simulink model "SPMSM_back_EMF_Observer_SMO_Trigger"  (R2022b)
settings: Solver=VariableStepAuto  StartTime=0.0  StopTime=4  FixedStep=1e-7  MaxStep=1e-7  RelTol=1e-6
undefined symbols (not defined in the file): DiscIntNeverNeededParam
libraries: slpidlib x4, dspsigops x4, dsparch4 x3, simulink x2, spsDCVoltageSourceLib x1, spsPermanentMagnetSynchronousMachineLib x1, dspstat3 x1, spsUniversalBridgeLib x1, spspowerguiLib x1
settings Model: Creator=SSC  LastModifiedBy=SSC

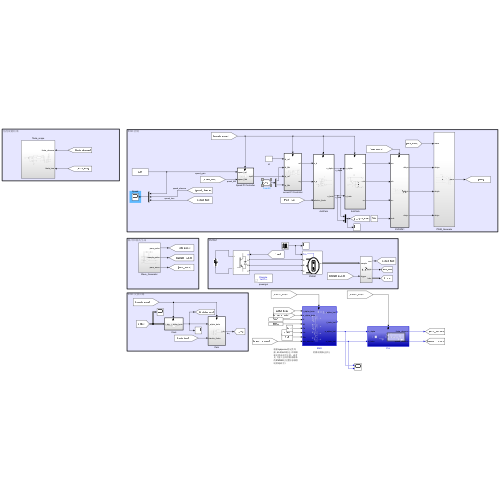
[thumbnail: Simulink's stored preview of the top-level diagram]
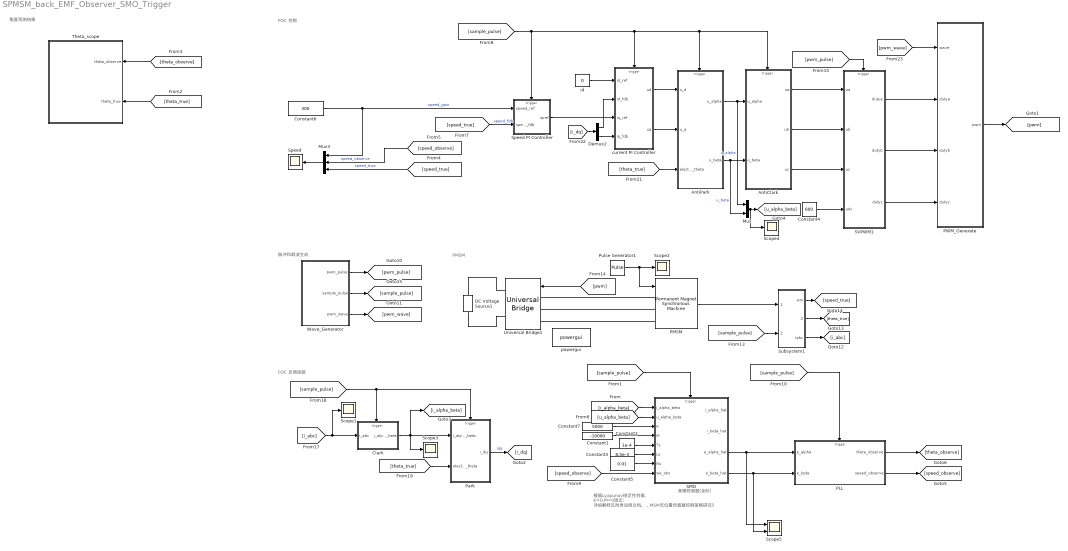
== system SPMSM_back_EMF_Observer_SMO_Trigger ==
  note: 根据Lyapunov稳定性判据, K>0,M<0稳定; 详细解释见附录说明文档。或者见《基于全阶滑模观测器的IPMSM无位置传感器控制策略研究》
  note: 滑模观测器(全阶)
  note: 角度观测结果
  note: FOC 控制
  note: FOC 反馈回路
  note: 脉冲和载波生成
  note: PMSM
  AntiClark : Subsystem
  AntiPark : Subsystem
  Clark : Subsystem
  Constant1 : Constant  Value=-10000
  Constant2 : Constant  Value=1e-4
  Constant3 : Constant  Value=8.5e-3
  Constant4 : Constant  Value=600
  Constant5 : Constant  Value=0.91
  Constant6 : Constant  Value=300
  Constant7 : Constant  Value=5000
  DC Voltage Source1 : spsDCVoltageSourceLib/DC Voltage Source  Amplitude=600  Measurements=None
  Demux2 : Demux  Outputs=2
  Mux : Mux  Inputs=2
  Mux3 : Mux  Inputs=3
  PLL : Subsystem  TreatAsAtomicUnit=on
  PMSM : spsPermanentMagnetSynchronousMachineLib/Permanent Magnet Synchronous Machine  NbPhases=3  FluxDistribution=Sinusoidal  RotorType=Round  MechanicalLoad=Torque Tm  PresetModel=No  ShowDetailedParameters=on  MeasurementBus=off  Resistance=0.91  Inductance=8.5e-3  dqInductances=[0.00396,0.00396]  La=8.5e-3  MachineConstant=Flux linkage established by magnets (V.s)  Flux=0.446  VoltageCst=161.7909  TorqueCst=1.338  Flat=120  Mechanical=[0.074 0.008 2 0]  PolePairs=4  InitialConditions=[300*2*pi/60,0,0,0]  InitialConditions5ph=[0 0 0 0 0 0]  RefAngle=Aligned with phase A axis (original Park)  IterativeDiscreteModel=Trapezoidal non iterative  TsBlock=-1  TsPowergui=0
  PWM_Generate : Subsystem
  Park : Subsystem
  Pulse Generator1 : DiscretePulseGenerator  PulseType=Time based  Period=3  PulseWidth=33.3  PhaseDelay=2.5
  SMO : Subsystem  TreatAsAtomicUnit=on
  SVPWM1 : Subsystem
  Scope{1..4} (4 alike) : Scope
  Scope5 : Scope  NumInputPorts=2
  Speed : Scope
  Speed PI Controller : Subsystem  TreatAsAtomicUnit=on
  Subsystem1 : Subsystem
  Theta_scope : Subsystem
  Universal Bridge1 : spsUniversalBridgeLib/Universal Bridge  Arms=3  SnubberResistance=1e5  SnubberCapacitance=inf  Device=IGBT / Diodes  Ron=1e-3  Lon=0  ForwardVoltages="[  0  0  ]"  ForwardVoltage=0  GTOparameters=[ 10e-6 , 20e-6 ]  IGBTparameters=[ 1e-6 , 2e-6 ]  Measurements=None  Measurements_2=None  converterType=Rectifier
  Wave_Generator : Subsystem
  current PI Controller : Subsystem
  id : Constant  Value=0
  powergui : spspowerguiLib/powergui  Priority=1  SimulationMode=Discrete  SampleTime=1e-7  frequency=60  Iterations=50  frequencyindice=0  Pbase=100e6  ErrMax=1e-4  UnitsV=kV  UnitsW=MW  buscounter=0  FunctionMessages=off  echomessages=off  EnableUseOfTLC=off  CurrentSourceSwitches=off  DisableSnubberDevices=off  DisableRonSwitches=off  DisableVfSwitches=off  DisplayEquations=off  AutomaticDiscreteSolvers=off  SolverType=Tustin/Backward Euler (TBE)  Interpol=off  ExternalGateDelay=off  methode=off  Ts=100  x0status=blocks  SPID=on  SwTol=0  HookPort=off  NonlinearTolerance=1e-4  nMaxIteration=100  ContinueOnMaxIteration=off  RestoreLinks=warning  ResistiveCurrentMeasurement=off  Frange=[0:2:500]  Ylog=off  Xlog=on  ShowGrid=off  save=off  variable=ZData  structure=0  ZoomFFT=off  StartTime=0.0  cycles=1  DisplayStyle=1  fundamental=60  FreqAxis=off  MaxFrequency=1000  frequencyindicesteady=1  RmsSteady=1  display=off
  wires:
  PMSM/1 -> Subsystem1/1(sample)
  [pwm] -> Universal Bridge1/1
  Subsystem1/2(theta) -> [theta_true]
  Subsystem1/3(Iabc) -> [i_abc]
  Pulse Generator1/1 -> PMSM/1, Scope2/1
  Wave_Generator/1(pwm_pulse) -> [pwm_pulse]
  Wave_Generator/2(sample_pulse) -> [sample_pulse]
  Wave_Generator/3(pwm_wave) -> [pwm_wave]
  Subsystem1/1(wm) -> [speed_true]
  [sample_pulse] -> Subsystem1/2(trigger)
  [sample_pulse] -> Park/Trigger, Clark/Trigger
  [theta_true] -> Park/2(electric_theta)
  Park/1(i_dq) -> [i_dq]  "idq"
  [i_abc] -> Scope1/1, Clark/1(i_abc)
  Clark/1(i_alpha_beta) -> [i_alpha_beta], Scope3/1, Park/1(i_alpha_beta)
  AntiClark/3(uc) -> SVPWM1/3(uc)
  [pwm_pulse] -> SVPWM1/Trigger
  AntiClark/1(ua) -> SVPWM1/1(ua)
  AntiClark/2(ub) -> SVPWM1/2(ub)
  SVPWM1/2(dutyb) -> PWM_Generate/3(dutyb)
  Constant4/1 -> SVPWM1/4(udc)
  SVPWM1/1(dutya) -> PWM_Generate/2(dutya)
  PWM_Generate/1(pwm) -> [pwm]
  SVPWM1/3(dutyc) -> PWM_Generate/4(dutyc)
  [pwm_wave] -> PWM_Generate/1(wave)
  [i_dq] -> Demux2/1
  id/1 -> current PI Controller/1(id_ref)
  Demux2/1 -> current PI Controller/2(id_fdb)
  Demux2/2 -> current PI Controller/4(iq_fdb)
  Speed PI Controller/1(iqref) -> current PI Controller/3(iq_ref)
  current PI Controller/1(ud) -> AntiPark/1(u_d)
  [theta_true] -> AntiPark/3(electric_theta)
  [speed_true] -> Speed PI Controller/2(speed_fdb)  "speed_fdb"
  current PI Controller/2(uq) -> AntiPark/2(u_q)
  AntiPark/1(u_alpha) -> Mux/1, AntiClark/1(u_alpha)  "u_alpha"
  AntiPark/2(u_beta) -> Mux/2, AntiClark/2(u_beta)  "u_beta"
  [theta_true] -> Theta_scope/2(theta_true)
  [theta_observe] -> Theta_scope/1(theta_observe)
  Constant6/1 -> Speed PI Controller/1(speed_ref), Mux3/1  "speed_gain"
  [speed_true] -> Mux3/3  "speed_true"
  [speed_observe] -> Mux3/2  "speed_observe"
  Mux3/1 -> Speed/1
  [sample_pulse] -> AntiClark/Trigger, AntiPark/Trigger, current PI Controller/Trigger, Speed PI Controller/Trigger
  Mux/1 -> Scope4/1, [u_alpha_beta]
  [i_alpha_beta] -> SMO/1(i_alpha_beta)
  [u_alpha_beta] -> SMO/2(u_alpha_beta)
  Constant7/1 -> SMO/3(K)
  Constant1/1 -> SMO/4(M)
  Constant2/1 -> SMO/5(Ts)
  Constant3/1 -> SMO/6(Ls)
  Constant5/1 -> SMO/7(Rs)
  [sample_pulse] -> SMO/Trigger
  SMO/3(e_alpha_hat) -> PLL/1(e_alpha), Scope5/1
  SMO/4(e_beta_hat) -> PLL/2(e_beta), Scope5/2
  [sample_pulse] -> PLL/Trigger
  PLL/2(speed_observe) -> [speed_observe]
  PLL/1(theta_observe) -> [theta_observe]
  [speed_observe] -> SMO/8(we_obs)
  connections:
  PMSM/LConn2 -- Universal Bridge1/LConn2
  PMSM/LConn1 -- Universal Bridge1/LConn1
  PMSM/LConn3 -- Universal Bridge1/LConn3
  Universal Bridge1/RConn1 -- DC Voltage Source1/RConn1
  DC Voltage Source1/LConn1 -- Universal Bridge1/RConn2

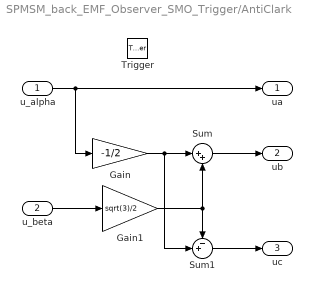
== system SPMSM_back_EMF_Observer_SMO_Trigger/AntiClark ==
  u_alpha : Inport
  u_beta : Inport  Port=2
  Trigger : TriggerPort  VariantControl=(inherit)
  Gain : Gain  Gain=-1/2
  Gain1 : Gain  Gain=sqrt(3)/2
  Sum : Sum  Inputs=|++
  Sum1 : Sum  Inputs=-+|
  ua : Outport
  ub : Outport  Port=2
  uc : Outport  Port=3
  wires:
  Sum1/1 -> uc/1
  Gain1/1 -> Sum1/1, Sum/2
  Sum/1 -> ub/1
  Gain/1 -> Sum/1, Sum1/2
  u_beta/1 -> Gain1/1
  u_alpha/1 -> ua/1, Gain/1

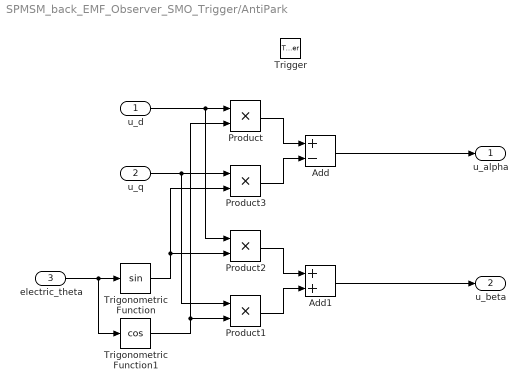
== system SPMSM_back_EMF_Observer_SMO_Trigger/AntiPark ==
  u_d : Inport
  u_q : Inport  Port=2
  electric_theta : Inport  Port=3
  Trigger : TriggerPort  VariantControl=(inherit)
  Add : Sum  Inputs=+-
  Add1 : Sum
  Product{,1..3} (4 alike) : Product
  Trigonometric Function : Trigonometry
  Trigonometric Function1 : Trigonometry  Operator=cos
  u_alpha : Outport
  u_beta : Outport  Port=2
  wires:
  electric_theta/1 -> Trigonometric Function1/1, Trigonometric Function/1
  u_d/1 -> Product2/1, Product/1
  Trigonometric Function1/1 -> Product/2, Product1/2
  u_q/1 -> Product1/1, Product3/1
  Trigonometric Function/1 -> Product2/2, Product3/2
  Product/1 -> Add/1
  Product3/1 -> Add/2
  Add/1 -> u_alpha/1
  Product2/1 -> Add1/1
  Product1/1 -> Add1/2
  Add1/1 -> u_beta/1

== system SPMSM_back_EMF_Observer_SMO_Trigger/Clark ==
  i_abc : Inport
  Trigger : TriggerPort  VariantControl=(inherit)
  Clark : Subsystem
  Demux : Demux  Outputs=3
  Mux6 : Mux  Inputs=2
  i_alpha_beta : Outport  VectorParamsAs1DForOutWhenUnconnected=off
  wires:
  Clark/2(I_beta) -> Mux6/2
  Mux6/1 -> i_alpha_beta/1
  Demux/3 -> Clark/3(I_c)
  Clark/1(I_alpha) -> Mux6/1
  i_abc/1 -> Demux/1
  Demux/2 -> Clark/2(I_b)
  Demux/1 -> Clark/1(I_a)

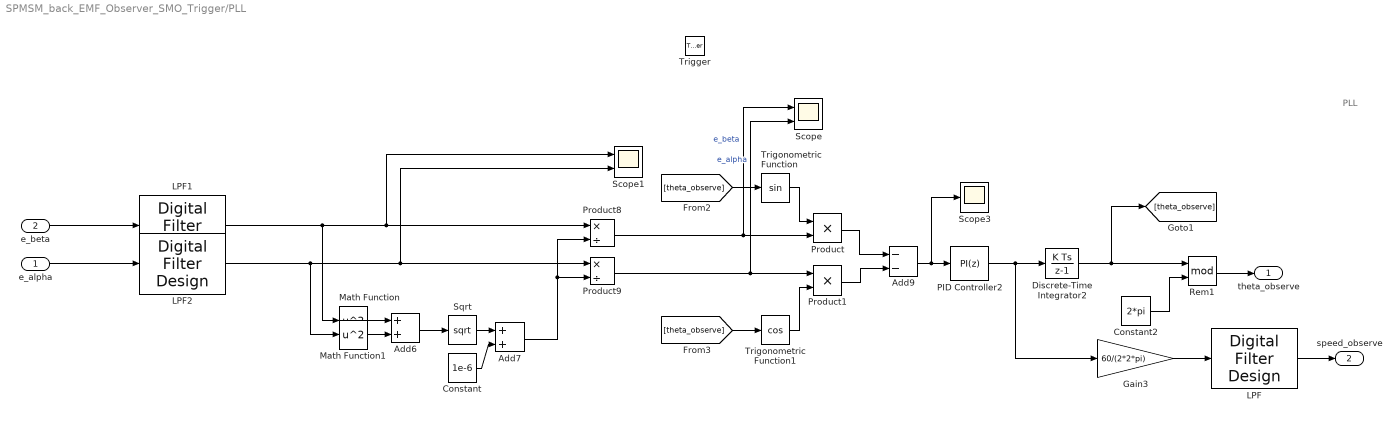
== system SPMSM_back_EMF_Observer_SMO_Trigger/PLL ==
  note: PLL
  e_alpha : Inport
  e_beta : Inport  Port=2
  Trigger : TriggerPort  VariantControl=(inherit)
  Add6 : Sum
  Add7 : Sum
  Add9 : Sum  Inputs=--
  Constant : Constant  Value=1e-6
  Constant2 : Constant  Value=2*pi
  Discrete-Time Integrator2 : DiscreteIntegrator  SampleTime=-1  ICPrevOutput=DiscIntNeverNeededParam  ICPrevScaledInput=DiscIntNeverNeededParam
  Gain3 : Gain  Gain=60/(2*2*pi)
  LPF : dsparch4/Digital Filter Design  mwdsp_browser_bugfix_var=off
  LPF1 : dsparch4/Digital Filter Design  mwdsp_browser_bugfix_var=off
  LPF2 : dsparch4/Digital Filter Design  mwdsp_browser_bugfix_var=off
  Math Function : Math  Operator=square
  Math Function1 : Math  Operator=square
  PID Controller2 : slpidlib/PID Controller  Controller=PI  Form=Parallel  TimeDomain=Discrete-time  UseExternalTs=off  SampleTime=-1  IntegratorMethod=Forward Euler  FilterMethod=Forward Euler  ControllerParametersSource=internal  P=10000  I=20000  UseKiTs=off  D=0  N=100  UseFilter=on  TunerSelectOption=Transfer Function Based (PID Tuner App)  InitialConditionSource=internal  InitialConditionForIntegrator=0  InitialConditionForFilter=0  DifferentiatorICPrevScaledInput=0  ExternalReset=none  TrackingMode=off  Kt=1  LimitOutput=off  SatLimitsSource=internal  UpperSaturationLimit=inf  LowerSaturationLimit=-inf  LinearizeAsGain=on  AntiWindupMode=none  Kb=1  LimitIntegrator=off  UpperIntegratorSaturationLimit=inf  LowerIntegratorSaturationLimit=-inf  POutMin=[]  POutMax=[]  IOutMin=[]  IOutMax=[]  DOutMin=[]  DOutMax=[]  NOutMin=[]  NOutMax=[]  SumOutMin=[]  SumOutMax=[]  SaturationOutMin=[]  SaturationOutMax=[]  PParamMin=[]  PParamMax=[]  IParamMin=[]  IParamMax=[]  DParamMin=[]  DParamMax=[]  NParamMin=[]  NParamMax=[]  KbParamMin=[]  KbParamMax=[]  KtParamMin=[]  KtParamMax=[]  KbOutMin=[]  KbOutMax=[]  KtOutMin=[]  KtOutMax=[]  IntegratorOutMin=[]  IntegratorOutMax=[]  FilterOutMin=[]  FilterOutMax=[]  SumI1OutMin=[]  SumI1OutMax=[]  SumI2OutMin=[]  SumI2OutMax=[]  SumI3OutMin=[]  SumI3OutMax=[]  SumI4OutMin=[]  SumI4OutMax=[]  SumDOutMin=[]  SumDOutMax=[]  DifferentiatorOutMin=[]  DifferentiatorOutMax=[]  FilterDiffOutCoefMin=[]  FilterDiffOutCoefMax=[]  ReciprocalOutMin=[]  ReciprocalOutMax=[]  SumDenOutMin=[]  SumDenOutMax=[]  SumNumOutMin=[]  SumNumOutMax=[]  DivideOutMin=[]  DivideOutMax=[]  UdiffTsProdOutMin=[]  UdiffTsProdOutMax=[]  NTsProdOutMin=[]  NTsProdOutMax=[]  UintegralTsProdOutMin=[]  UintegralTsProdOutMax=[]  UngainTsProdOutMin=[]  UngainTsProdOutMax=[]  ClampingZeroOutDataTypeStr=Inherit: Inherit via back propagation  ClampingZeroOutMin=[]  ClampingZeroOutMax=[]  FilterDenConstantOutDataTypeStr=Inherit: Inherit via back propagation  FilterDenConstantOutMin=[]  FilterDenConstantOutMax=[]  PCopyOutDataTypeStr=Inherit: Inherit via back propagation  PCopyOutMin=[]  PCopyOutMax=[]  NCopyOutDataTypeStr=Inherit: Inherit via back propagation  NCopyOutMin=[]  NCopyOutMax=[]  IntegratorContinuousStateAttributes=''  IntegratorStateMustResolveToSignalObject=off  IntegratorRTWStateStorageClass=Auto  FilterContinuousStateAttributes=''  FilterStateMustResolveToSignalObject=off  FilterRTWStateStorageClass=Auto  ParallelPVariant=InternalParameters  IdealPVariant=Disabled  IVariant=InternalParameters  DVariant=Disabled  IntegratorVariant=Discrete  SatVariant=Disabled  AWVariant=Passthrough  PCopyVariant=Disabled  TRVariant=Disabled  FdbkBlocksVariant=Forward  IdealPFdbkVariant=Disabled  SatFdbkVariant=Disabled  DerivativeFilterVariant=Disabled  NVariant=Disabled  NCopyVariant=Disabled_SignalSpec  FilterICVariant=Disabled  IntegratorICVariant=InternalICs  ExternalResetVariant=Disabled  TRSumVariant=Passthrough  SumFdbkVariant=Disabled  SumVariant=Sum_PI  TsampFilterVariant=InternalTs  TsampNgainVariant=Passthrough  TsampIntegralVariant=Passthrough  ExternalSaturationOutDataTypeStr=Inherit: Same as second input
  Product : Product
  Product1 : Product
  Product8 : Product  Inputs=*/
  Product9 : Product  Inputs=*/
  Rem1 : Math  Operator=mod
  Scope : Scope  NumInputPorts=2
  Scope1 : Scope  NumInputPorts=2
  Scope3 : Scope
  Sqrt : Sqrt
  Trigonometric Function : Trigonometry
  Trigonometric Function1 : Trigonometry  Operator=cos
  theta_observe : Outport
  speed_observe : Outport  Port=2  VectorParamsAs1DForOutWhenUnconnected=off
  wires:
  Trigonometric Function1/1 -> Product1/2
  [theta_observe] -> Trigonometric Function1/1
  Rem1/1 -> theta_observe/1
  Constant/1 -> Add7/2
  Product9/1 -> Scope/2, Product1/1  "e_alpha"
  Add7/1 -> Product8/2, Product9/2
  Sqrt/1 -> Add7/1
  Add6/1 -> Sqrt/1
  Math Function/1 -> Add6/1
  Math Function1/1 -> Add6/2
  LPF/1 -> speed_observe/1
  Gain3/1 -> LPF/1
  [theta_observe] -> Trigonometric Function/1
  Product1/1 -> Add9/2
  Discrete-Time Integrator2/1 -> Rem1/1, [theta_observe]
  Product8/1 -> Product/2, Scope/1  "e_beta"
  Constant2/1 -> Rem1/2
  Product/1 -> Add9/1
  Trigonometric Function/1 -> Product/1
  Add9/1 -> Scope3/1, PID Controller2/1
  PID Controller2/1 -> Gain3/1, Discrete-Time Integrator2/1
  e_beta/1 -> LPF1/1
  e_alpha/1 -> LPF2/1
  LPF1/1 -> Math Function/1, Product8/1, Scope1/1
  LPF2/1 -> Math Function1/1, Product9/1, Scope1/2

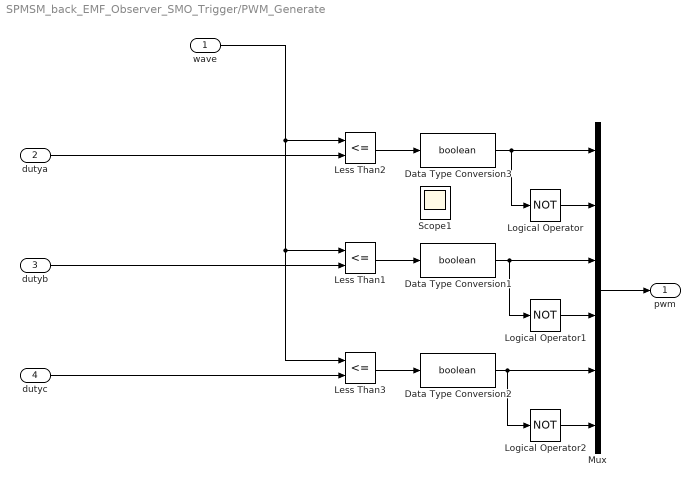
== system SPMSM_back_EMF_Observer_SMO_Trigger/PWM_Generate ==
  wave : Inport
  dutya : Inport  Port=2
  dutyb : Inport  Port=3
  dutyc : Inport  Port=4
  Data Type Conversion1 : DataTypeConversion  OutDataTypeStr=boolean  SaturateOnIntegerOverflow=off  RndMeth=Floor
  Data Type Conversion2 : DataTypeConversion  OutDataTypeStr=boolean  SaturateOnIntegerOverflow=off  RndMeth=Floor
  Data Type Conversion3 : DataTypeConversion  OutDataTypeStr=boolean  SaturateOnIntegerOverflow=off  RndMeth=Floor
  Less Than1 : RelationalOperator  Operator=<=  OutDataTypeStr=boolean  RndMeth=Simplest  InputSameDT=off
  Less Than2 : RelationalOperator  Operator=<=  OutDataTypeStr=boolean  RndMeth=Simplest  InputSameDT=off
  Less Than3 : RelationalOperator  Operator=<=  OutDataTypeStr=boolean  RndMeth=Simplest  InputSameDT=off
  Logical Operator : Logic  Operator=NOT  AllPortsSameDT=off  OutDataTypeStr=boolean
  Logical Operator1 : Logic  Operator=NOT  AllPortsSameDT=off  OutDataTypeStr=boolean
  Logical Operator2 : Logic  Operator=NOT  AllPortsSameDT=off  OutDataTypeStr=boolean
  Mux : Mux  Inputs=6
  Scope1 : Scope  NumInputPorts=2
  pwm : Outport
  wires:
  wave/1 -> Less Than3/1, Less Than1/1, Less Than2/1
  Less Than1/1 -> Data Type Conversion1/1
  Less Than2/1 -> Data Type Conversion3/1
  dutyb/1 -> Less Than1/2
  Less Than3/1 -> Data Type Conversion2/1
  dutya/1 -> Less Than2/2
  dutyc/1 -> Less Than3/2
  Data Type Conversion3/1 -> Logical Operator/1, Mux/1
  Logical Operator/1 -> Mux/2
  Data Type Conversion1/1 -> Logical Operator1/1, Mux/3
  Data Type Conversion2/1 -> Logical Operator2/1, Mux/5
  Logical Operator2/1 -> Mux/6
  Mux/1 -> pwm/1
  Logical Operator1/1 -> Mux/4

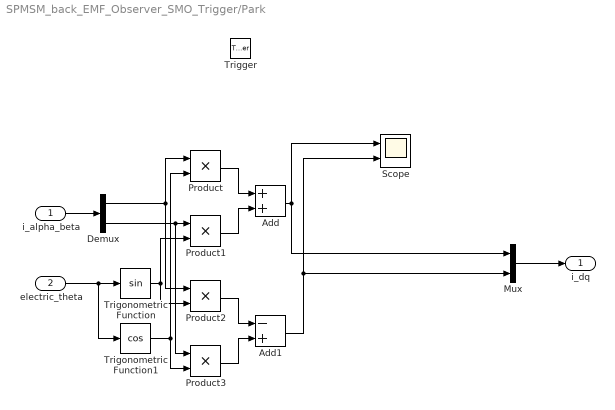
== system SPMSM_back_EMF_Observer_SMO_Trigger/Park ==
  i_alpha_beta : Inport
  electric_theta : Inport  Port=2
  Trigger : TriggerPort  VariantControl=(inherit)
  Add : Sum
  Add1 : Sum  Inputs=-+
  Demux : Demux  Outputs=2
  Mux : Mux  Inputs=2
  Product{,1..3} (4 alike) : Product
  Scope : Scope  NumInputPorts=2
  Trigonometric Function : Trigonometry
  Trigonometric Function1 : Trigonometry  Operator=cos
  i_dq : Outport
  wires:
  electric_theta/1 -> Trigonometric Function1/1, Trigonometric Function/1
  Trigonometric Function1/1 -> Product3/2, Product/2
  Demux/2 -> Product3/1, Product1/1
  Trigonometric Function/1 -> Product2/2, Product1/2
  Product/1 -> Add/1
  Product1/1 -> Add/2
  Product2/1 -> Add1/1
  Product3/1 -> Add1/2
  Demux/1 -> Product/1, Product2/1
  i_alpha_beta/1 -> Demux/1
  Mux/1 -> i_dq/1
  Add/1 -> Mux/1, Scope/1
  Add1/1 -> Mux/2, Scope/2

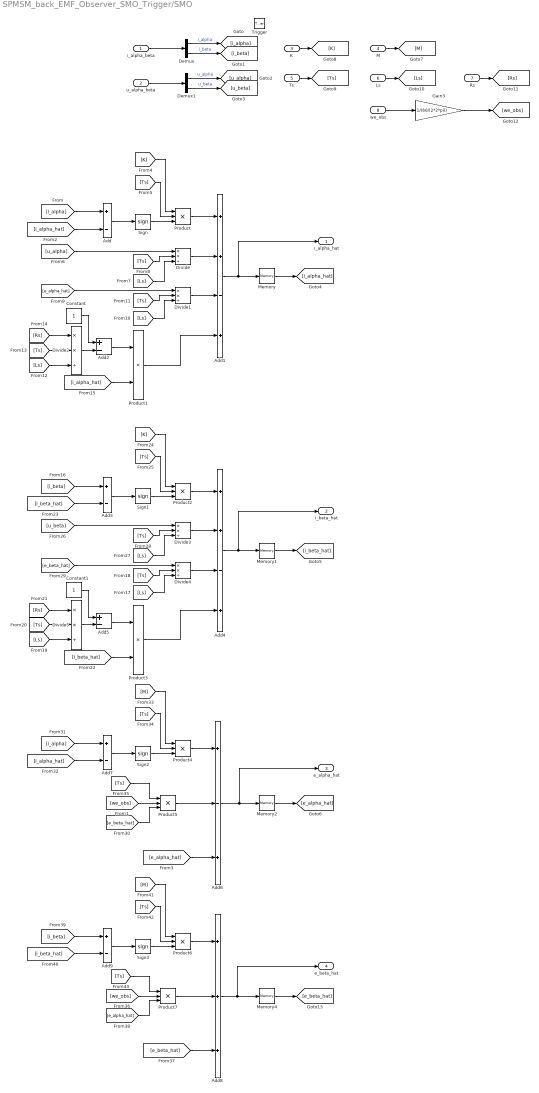
== system SPMSM_back_EMF_Observer_SMO_Trigger/SMO ==
  i_alpha_beta : Inport
  u_alpha_beta : Inport  Port=2
  K : Inport  Port=3
  M : Inport  Port=4
  Ts : Inport  Port=5
  Ls : Inport  Port=6
  Rs : Inport  Port=7
  we_obs : Inport  Port=8  LatchByDelayingOutsideSignal=on
  Trigger : TriggerPort  VariantControl=(inherit)
  Add{,2..3,5,7,9} (6 alike) : Sum  Inputs=+-
  Add1 : Sum  Inputs=++-+
  Add4 : Sum  Inputs=++-+
  Add6 : Sum  Inputs=+-+
  Add8 : Sum  Inputs=+++
  Constant : Constant
  Constant1 : Constant
  Demux : Demux  Outputs=2
  Demux1 : Demux  Outputs=2
  Divide{,1..5} (6 alike) : Product  Inputs=**/
  Gain3 : Gain  Gain=1/(60/(2*2*pi))
  Memory{,1..2,4} (4 alike) : Memory  InheritSampleTime=on
  Product{,2,4..7} (6 alike) : Product  Inputs=3
  Product1 : Product
  Product3 : Product
  Sign{,1..3} (4 alike) : Signum
  i_alpha_hat : Outport
  i_beta_hat : Outport  Port=2
  e_alpha_hat : Outport  Port=3
  e_beta_hat : Outport  Port=4
  wires:
  i_alpha_beta/1 -> Demux/1
  Demux/1 -> [i_alpha]  "i_alpha"
  Demux/2 -> [i_beta]  "i_beta"
  u_alpha_beta/1 -> Demux1/1
  Demux1/2 -> [u_beta]  "u_beta"
  Demux1/1 -> [u_alpha]  "u_alpha"
  [i_alpha] -> Add/1
  Memory/1 -> [i_alpha_hat]
  Memory1/1 -> [i_beta_hat]
  Memory2/1 -> [e_alpha_hat]
  [i_alpha_hat] -> Add/2
  Add/1 -> Sign/1
  Sign/1 -> Product/3
  K/1 -> [K]
  Ts/1 -> [Ts]
  [K] -> Product/1
  [Ts] -> Product/2
  Ls/1 -> [Ls]
  [Ls] -> Divide/3
  [u_alpha] -> Divide/1
  [Ts] -> Divide/2
  Product/1 -> Add1/1
  Divide/1 -> Add1/2
  [e_alpha_hat] -> Divide1/1
  [Ls] -> Divide1/3
  Divide1/1 -> Add1/3
  [Ts] -> Divide1/2
  Rs/1 -> [Rs]
  [Ls] -> Divide2/3
  [Ts] -> Divide2/2
  [Rs] -> Divide2/1
  Divide2/1 -> Add2/2
  Constant/1 -> Add2/1
  Add2/1 -> Product1/1
  [i_alpha_hat] -> Product1/2
  Product1/1 -> Add1/4
  [u_beta] -> Divide3/1
  Product3/1 -> Add4/4
  [i_beta_hat] -> Product3/2
  [Rs] -> Divide5/1
  [Ls] -> Divide4/3
  [e_beta_hat] -> Divide4/1
  [Ts] -> Divide4/2
  [Ts] -> Divide5/2
  [Ls] -> Divide3/3
  [Ls] -> Divide5/3
  Sign1/1 -> Product2/3
  [K] -> Product2/1
  [i_beta_hat] -> Add3/2
  Constant1/1 -> Add5/1
  Add5/1 -> Product3/1
  Product2/1 -> Add4/1
  Add3/1 -> Sign1/1
  [Ts] -> Product2/2
  Divide5/1 -> Add5/2
  Divide3/1 -> Add4/2
  [i_beta] -> Add3/1
  Divide4/1 -> Add4/3
  [Ts] -> Divide3/2
  Add1/1 -> i_alpha_hat/1, Memory/1
  [Ts] -> Product4/2
  Add7/1 -> Sign2/1
  [i_alpha] -> Add7/1
  [i_alpha_hat] -> Add7/2
  [M] -> Product4/1
  Sign2/1 -> Product4/3
  Product4/1 -> Add6/1
  [e_alpha_hat] -> Add6/3
  Product5/1 -> Add6/2
  [we_obs] -> Product5/2
  [e_beta_hat] -> Product5/3
  [Ts] -> Product5/1
  [e_beta_hat] -> Add8/3
  [Ts] -> Product7/1
  Product6/1 -> Add8/1
  Sign3/1 -> Product6/3
  [M] -> Product6/1
  Add9/1 -> Sign3/1
  [i_beta] -> Add9/1
  [i_beta_hat] -> Add9/2
  [we_obs] -> Product7/2
  [Ts] -> Product6/2
  [e_alpha_hat] -> Product7/3
  Add8/1 -> e_beta_hat/1, Memory4/1
  Product7/1 -> Add8/2
  Memory4/1 -> [e_beta_hat]
  Add4/1 -> i_beta_hat/1, Memory1/1
  Add6/1 -> e_alpha_hat/1, Memory2/1
  M/1 -> [M]
  we_obs/1 -> Gain3/1
  Gain3/1 -> [we_obs]

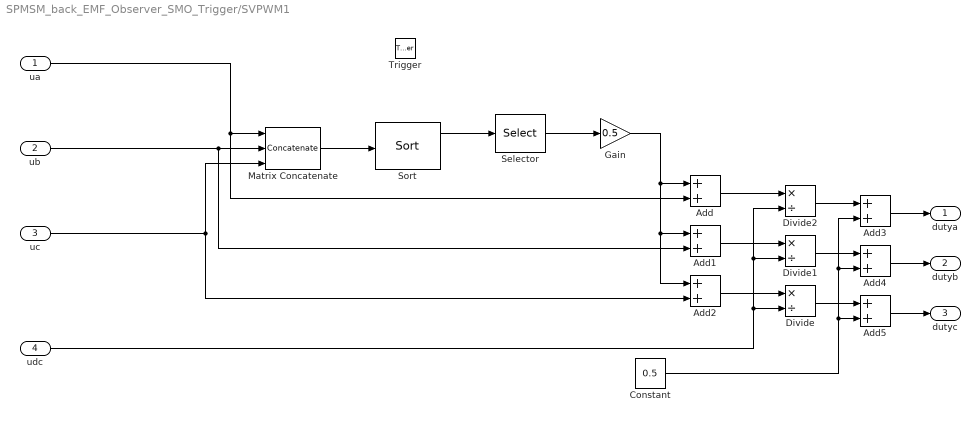
== system SPMSM_back_EMF_Observer_SMO_Trigger/SVPWM1 ==
  ua : Inport
  ub : Inport  Port=2
  uc : Inport  Port=3
  udc : Inport  Port=4
  Trigger : TriggerPort  VariantControl=(inherit)
  Add{,1..5} (6 alike) : Sum
  Constant : Constant  Value=0.5
  Divide : Product  Inputs=*/
  Divide1 : Product  Inputs=*/
  Divide2 : Product  Inputs=*/
  Gain : Gain  Gain=0.5
  Matrix Concatenate : Concatenate  NumInputs=3  ConcatenateDimension=2
  Selector : Selector  InputPortWidth=3  IndexOptions=Index vector (dialog)  Indices=2  OutputSizes=1
  Sort : dspstat3/Sort  otype=Value and Index  dir=Ascending  sortAlg=Quick sort  roundingMode=Floor  overflowMode=off  accumDataTypeStr=Inherit: Same as product output  accumLastDataTypeStr=Inherit: Same as product output
  dutya : Outport
  dutyb : Outport  Port=2
  dutyc : Outport  Port=3
  wires:
  Selector/1 -> Gain/1
  udc/1 -> Divide/2, Divide2/2, Divide1/2
  Add1/1 -> Divide1/1
  Sort/1 -> Selector/1
  Matrix Concatenate/1 -> Sort/1
  Add2/1 -> Divide/1
  Gain/1 -> Add2/1, Add1/1, Add/1
  ua/1 -> Add/2, Matrix Concatenate/1
  Add/1 -> Divide2/1
  uc/1 -> Matrix Concatenate/3, Add2/2
  ub/1 -> Add1/2, Matrix Concatenate/2
  Divide2/1 -> Add3/1
  Divide1/1 -> Add4/1
  Divide/1 -> Add5/1
  Constant/1 -> Add5/2, Add4/2, Add3/2
  Add3/1 -> dutya/1
  Add4/1 -> dutyb/1
  Add5/1 -> dutyc/1

== system SPMSM_back_EMF_Observer_SMO_Trigger/Speed PI Controller ==
  speed_ref : Inport
  speed_fdb : Inport  Port=2
  Trigger : TriggerPort  VariantControl=(inherit)
  Speed PI Controller : slpidlib/PID Controller  Controller=PI  Form=Parallel  TimeDomain=Discrete-time  UseExternalTs=off  SampleTime=-1  IntegratorMethod=Forward Euler  FilterMethod=Forward Euler  ControllerParametersSource=internal  P=3.786/30  I=44.84/30/2  UseKiTs=off  D=0  N=100  UseFilter=on  TunerSelectOption=Transfer Function Based (PID Tuner App)  InitialConditionSource=internal  InitialConditionForIntegrator=0  InitialConditionForFilter=0  DifferentiatorICPrevScaledInput=0  ExternalReset=none  TrackingMode=off  Kt=1  LimitOutput=off  SatLimitsSource=internal  UpperSaturationLimit=5.65  LowerSaturationLimit=-5.65  LinearizeAsGain=on  AntiWindupMode=clamping  Kb=1  LimitIntegrator=off  UpperIntegratorSaturationLimit=inf  LowerIntegratorSaturationLimit=-inf  POutMin=[]  POutMax=[]  IOutMin=[]  IOutMax=[]  DOutMin=[]  DOutMax=[]  NOutMin=[]  NOutMax=[]  SumOutMin=[]  SumOutMax=[]  SaturationOutMin=[]  SaturationOutMax=[]  PParamMin=[]  PParamMax=[]  IParamMin=[]  IParamMax=[]  DParamMin=[]  DParamMax=[]  NParamMin=[]  NParamMax=[]  KbParamMin=[]  KbParamMax=[]  KtParamMin=[]  KtParamMax=[]  KbOutMin=[]  KbOutMax=[]  KtOutMin=[]  KtOutMax=[]  IntegratorOutMin=[]  IntegratorOutMax=[]  FilterOutMin=[]  FilterOutMax=[]  SumI1OutMin=[]  SumI1OutMax=[]  SumI2OutMin=[]  SumI2OutMax=[]  SumI3OutMin=[]  SumI3OutMax=[]  SumI4OutMin=[]  SumI4OutMax=[]  SumDOutMin=[]  SumDOutMax=[]  DifferentiatorOutMin=[]  DifferentiatorOutMax=[]  FilterDiffOutCoefMin=[]  FilterDiffOutCoefMax=[]  ReciprocalOutMin=[]  ReciprocalOutMax=[]  SumDenOutMin=[]  SumDenOutMax=[]  SumNumOutMin=[]  SumNumOutMax=[]  DivideOutMin=[]  DivideOutMax=[]  UdiffTsProdOutMin=[]  UdiffTsProdOutMax=[]  NTsProdOutMin=[]  NTsProdOutMax=[]  UintegralTsProdOutMin=[]  UintegralTsProdOutMax=[]  UngainTsProdOutMin=[]  UngainTsProdOutMax=[]  ClampingZeroOutDataTypeStr=Inherit: Inherit via back propagation  ClampingZeroOutMin=[]  ClampingZeroOutMax=[]  FilterDenConstantOutDataTypeStr=Inherit: Inherit via back propagation  FilterDenConstantOutMin=[]  FilterDenConstantOutMax=[]  PCopyOutDataTypeStr=Inherit: Inherit via back propagation  PCopyOutMin=[]  PCopyOutMax=[]  NCopyOutDataTypeStr=Inherit: Inherit via back propagation  NCopyOutMin=[]  NCopyOutMax=[]  IntegratorContinuousStateAttributes=''  IntegratorStateMustResolveToSignalObject=off  IntegratorRTWStateStorageClass=Auto  FilterContinuousStateAttributes=''  FilterStateMustResolveToSignalObject=off  FilterRTWStateStorageClass=Auto  ParallelPVariant=InternalParameters  IdealPVariant=Disabled  IVariant=InternalParameters  DVariant=Disabled  IntegratorVariant=Discrete  SatVariant=Disabled  AWVariant=Passthrough  PCopyVariant=Disabled  TRVariant=Disabled  FdbkBlocksVariant=Forward  IdealPFdbkVariant=Disabled  SatFdbkVariant=Disabled  DerivativeFilterVariant=Disabled  NVariant=Disabled  NCopyVariant=Disabled_SignalSpec  FilterICVariant=Disabled  IntegratorICVariant=InternalICs  ExternalResetVariant=Disabled  TRSumVariant=Passthrough  SumFdbkVariant=Disabled  SumVariant=Sum_PI  TsampFilterVariant=InternalTs  TsampNgainVariant=Passthrough  TsampIntegralVariant=Passthrough  ExternalSaturationOutDataTypeStr=Inherit: Same as second input
  Sum3 : Sum  Inputs=|+-
  iqref : Outport
  wires:
  Sum3/1 -> Speed PI Controller/1
  Speed PI Controller/1 -> iqref/1
  speed_ref/1 -> Sum3/1
  speed_fdb/1 -> Sum3/2

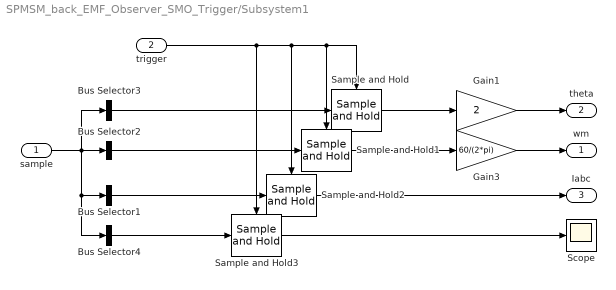
== system SPMSM_back_EMF_Observer_SMO_Trigger/Subsystem1 ==
  sample : Inport
  trigger : Inport  Port=2
  Bus Selector1 : BusSelector  OutputSignals=Stator current is_a (A),Stator current is_b (A),Stator current is_c (A)  OutputAsBus=on
  Bus Selector2 : BusSelector  OutputSignals=Rotor speed wm (rad/s)  OutputAsBus=on
  Bus Selector3 : BusSelector  OutputSignals=Rotor angle thetam (rad)  OutputAsBus=on
  Bus Selector4 : BusSelector  OutputSignals=Rotor speed wm (rad/s)  OutputAsBus=on
  Gain1 : Gain  Gain=2
  Gain3 : Gain  Gain=60/(2*pi)
  Sample and Hold{,1..3} (4 alike) : dspsigops/Sample and Hold  trig=Rising edge  initCond=0  latchinput=off
  Scope : Scope
  wm : Outport  VectorParamsAs1DForOutWhenUnconnected=off
  theta : Outport  Port=2  VectorParamsAs1DForOutWhenUnconnected=off
  Iabc : Outport  Port=3  VectorParamsAs1DForOutWhenUnconnected=off
  wires:
  sample/1 -> Bus Selector4/1, Bus Selector1/1, Bus Selector3/1, Bus Selector2/1
  Gain1/1 -> theta/1
  Sample and Hold/1 -> Gain1/1
  Bus Selector3/1 -> Sample and Hold/1
  Bus Selector2/1 -> Sample and Hold1/1
  Bus Selector1/1 -> Sample and Hold2/1
  Sample and Hold2/1 -> Iabc/1
  Bus Selector4/1 -> Sample and Hold3/1
  Sample and Hold3/1 -> Scope/1
  trigger/1 -> Sample and Hold3/Trigger, Sample and Hold2/Trigger, Sample and Hold1/Trigger, Sample and Hold/Trigger
  Sample and Hold1/1 -> Gain3/1
  Gain3/1 -> wm/1

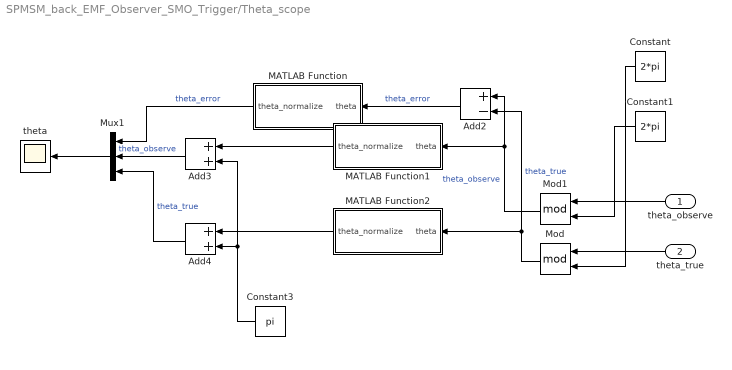
== system SPMSM_back_EMF_Observer_SMO_Trigger/Theta_scope ==
  theta_observe : Inport
  theta_true : Inport  Port=2
  Add2 : Sum  Inputs=+-
  Add3 : Sum
  Add4 : Sum
  Constant : Constant  Value=2*pi
  Constant1 : Constant  Value=2*pi
  Constant3 : Constant  Value=pi
  MATLAB Function : MATLAB Function  TreatAsAtomicUnit=on
  MATLAB Function1 : MATLAB Function  TreatAsAtomicUnit=on
  MATLAB Function2 : MATLAB Function  TreatAsAtomicUnit=on
  Mod : Math  Operator=mod  SignedPower=on
  Mod1 : Math  Operator=mod  SignedPower=on
  Mux1 : Mux  Inputs=3
  theta : Scope
  wires:
  Add4/1 -> Mux1/3  "theta_true"
  Constant1/1 -> Mod1/2
  Constant/1 -> Mod/2
  MATLAB Function2/1(theta_normalize) -> Add4/1
  Mod/1 -> Add2/2, MATLAB Function2/1(theta)  "theta_true"
  Mux1/1 -> theta/1
  theta_observe/1 -> Mod1/1
  Constant3/1 -> Add4/2, Add3/2
  MATLAB Function/1(theta_normalize) -> Mux1/1  "theta_error"
  MATLAB Function1/1(theta_normalize) -> Add3/1
  Mod1/1 -> Add2/1, MATLAB Function1/1(theta)  "theta_observe"
  Add3/1 -> Mux1/2  "theta_observe"
  Add2/1 -> MATLAB Function/1(theta)  "theta_error"
  theta_true/1 -> Mod/1

== system SPMSM_back_EMF_Observer_SMO_Trigger/Wave_Generator ==
  Constant : Constant  Value=1e-6
  Less Than1 : RelationalOperator  Operator=<=  OutDataTypeStr=boolean  RndMeth=Simplest  InputSameDT=off
  Less Than2 : RelationalOperator  Operator=<=  OutDataTypeStr=boolean  RndMeth=Simplest  InputSameDT=off
  Scope1 : Scope  NumInputPorts=2
  Scope2 : Scope  NumInputPorts=2
  载波 : simulink/Sources/Repeating Sequence  rep_seq_t=[0 0.5e-4 1e-4]  rep_seq_y=[0 1 0]
  载波_反向 : simulink/Sources/Repeating Sequence  rep_seq_t=[0 0.5e-4 1e-4]  rep_seq_y=[1 0 1]
  pwm_pulse : Outport
  sample_pulse : Outport  Port=2
  pwm_wave : Outport  Port=3
  wires:
  Less Than2/1 -> pwm_pulse/1, Scope1/1  "pwm_pulse"
  Constant/1 -> Less Than1/2, Less Than2/2
  载波/1 -> pwm_wave/1, Less Than2/1, Scope2/1  "wave"
  Less Than1/1 -> sample_pulse/1, Scope1/2  "sample_pulse"
  载波_反向/1 -> Scope2/2, Less Than1/1  "wave_inv"

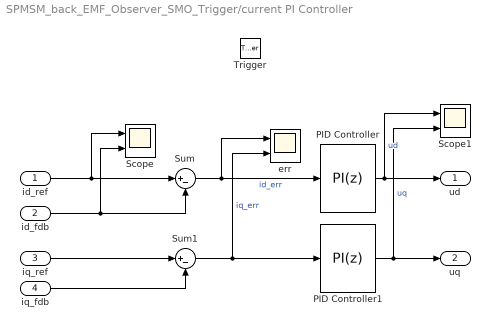
== system SPMSM_back_EMF_Observer_SMO_Trigger/current PI Controller ==
  id_ref : Inport
  id_fdb : Inport  Port=2
  iq_ref : Inport  Port=3
  iq_fdb : Inport  Port=4
  Trigger : TriggerPort  VariantControl=(inherit)
  PID Controller : slpidlib/PID Controller  Controller=PI  Form=Parallel  TimeDomain=Discrete-time  UseExternalTs=off  SampleTime=-1  IntegratorMethod=Forward Euler  FilterMethod=Forward Euler  ControllerParametersSource=internal  P=19.8  I=4550  UseKiTs=off  D=0  N=100  UseFilter=on  TunerSelectOption=Transfer Function Based (PID Tuner App)  InitialConditionSource=internal  InitialConditionForIntegrator=0  InitialConditionForFilter=0  DifferentiatorICPrevScaledInput=0  ExternalReset=none  TrackingMode=off  Kt=1  LimitOutput=on  SatLimitsSource=internal  UpperSaturationLimit=600/sqrt(3)  LowerSaturationLimit=-600/sqrt(3)  LinearizeAsGain=on  AntiWindupMode=clamping  Kb=1  LimitIntegrator=off  UpperIntegratorSaturationLimit=inf  LowerIntegratorSaturationLimit=-inf  POutMin=[]  POutMax=[]  IOutMin=[]  IOutMax=[]  DOutMin=[]  DOutMax=[]  NOutMin=[]  NOutMax=[]  SumOutMin=[]  SumOutMax=[]  SaturationOutMin=[]  SaturationOutMax=[]  PParamMin=[]  PParamMax=[]  IParamMin=[]  IParamMax=[]  DParamMin=[]  DParamMax=[]  NParamMin=[]  NParamMax=[]  KbParamMin=[]  KbParamMax=[]  KtParamMin=[]  KtParamMax=[]  KbOutMin=[]  KbOutMax=[]  KtOutMin=[]  KtOutMax=[]  IntegratorOutMin=[]  IntegratorOutMax=[]  FilterOutMin=[]  FilterOutMax=[]  SumI1OutMin=[]  SumI1OutMax=[]  SumI2OutMin=[]  SumI2OutMax=[]  SumI3OutMin=[]  SumI3OutMax=[]  SumI4OutMin=[]  SumI4OutMax=[]  SumDOutMin=[]  SumDOutMax=[]  DifferentiatorOutMin=[]  DifferentiatorOutMax=[]  FilterDiffOutCoefMin=[]  FilterDiffOutCoefMax=[]  ReciprocalOutMin=[]  ReciprocalOutMax=[]  SumDenOutMin=[]  SumDenOutMax=[]  SumNumOutMin=[]  SumNumOutMax=[]  DivideOutMin=[]  DivideOutMax=[]  UdiffTsProdOutMin=[]  UdiffTsProdOutMax=[]  NTsProdOutMin=[]  NTsProdOutMax=[]  UintegralTsProdOutMin=[]  UintegralTsProdOutMax=[]  UngainTsProdOutMin=[]  UngainTsProdOutMax=[]  ClampingZeroOutDataTypeStr=Inherit: Inherit via back propagation  ClampingZeroOutMin=[]  ClampingZeroOutMax=[]  FilterDenConstantOutDataTypeStr=Inherit: Inherit via back propagation  FilterDenConstantOutMin=[]  FilterDenConstantOutMax=[]  PCopyOutDataTypeStr=Inherit: Inherit via back propagation  PCopyOutMin=[]  PCopyOutMax=[]  NCopyOutDataTypeStr=Inherit: Inherit via back propagation  NCopyOutMin=[]  NCopyOutMax=[]  IntegratorContinuousStateAttributes=''  IntegratorStateMustResolveToSignalObject=off  IntegratorRTWStateStorageClass=Auto  FilterContinuousStateAttributes=''  FilterStateMustResolveToSignalObject=off  FilterRTWStateStorageClass=Auto  ParallelPVariant=InternalParameters  IdealPVariant=Disabled  IVariant=InternalParameters  DVariant=Disabled  IntegratorVariant=Discrete  SatVariant=Enabled  AWVariant=DiscClampingParallel  PCopyVariant=Disabled  TRVariant=Disabled  FdbkBlocksVariant=Forward  IdealPFdbkVariant=Disabled  SatFdbkVariant=Disabled  DerivativeFilterVariant=Disabled  NVariant=Disabled  NCopyVariant=Disabled_SignalSpec  FilterICVariant=Disabled  IntegratorICVariant=InternalICs  ExternalResetVariant=Disabled  TRSumVariant=Passthrough  SumFdbkVariant=Disabled  SumVariant=Sum_PI  TsampFilterVariant=InternalTs  TsampNgainVariant=Passthrough  TsampIntegralVariant=Passthrough  ExternalSaturationOutDataTypeStr=Inherit: Same as second input
  PID Controller1 : slpidlib/PID Controller  Controller=PI  Form=Parallel  TimeDomain=Discrete-time  UseExternalTs=off  SampleTime=-1  IntegratorMethod=Forward Euler  FilterMethod=Forward Euler  ControllerParametersSource=internal  P=19.8  I=4550  UseKiTs=off  D=0  N=100  UseFilter=on  TunerSelectOption=Transfer Function Based (PID Tuner App)  InitialConditionSource=internal  InitialConditionForIntegrator=0  InitialConditionForFilter=0  DifferentiatorICPrevScaledInput=0  ExternalReset=none  TrackingMode=off  Kt=1  LimitOutput=on  SatLimitsSource=internal  UpperSaturationLimit=600/sqrt(3)  LowerSaturationLimit=-600/sqrt(3)  LinearizeAsGain=on  AntiWindupMode=clamping  Kb=1  LimitIntegrator=off  UpperIntegratorSaturationLimit=inf  LowerIntegratorSaturationLimit=-inf  POutMin=[]  POutMax=[]  IOutMin=[]  IOutMax=[]  DOutMin=[]  DOutMax=[]  NOutMin=[]  NOutMax=[]  SumOutMin=[]  SumOutMax=[]  SaturationOutMin=[]  SaturationOutMax=[]  PParamMin=[]  PParamMax=[]  IParamMin=[]  IParamMax=[]  DParamMin=[]  DParamMax=[]  NParamMin=[]  NParamMax=[]  KbParamMin=[]  KbParamMax=[]  KtParamMin=[]  KtParamMax=[]  KbOutMin=[]  KbOutMax=[]  KtOutMin=[]  KtOutMax=[]  IntegratorOutMin=[]  IntegratorOutMax=[]  FilterOutMin=[]  FilterOutMax=[]  SumI1OutMin=[]  SumI1OutMax=[]  SumI2OutMin=[]  SumI2OutMax=[]  SumI3OutMin=[]  SumI3OutMax=[]  SumI4OutMin=[]  SumI4OutMax=[]  SumDOutMin=[]  SumDOutMax=[]  DifferentiatorOutMin=[]  DifferentiatorOutMax=[]  FilterDiffOutCoefMin=[]  FilterDiffOutCoefMax=[]  ReciprocalOutMin=[]  ReciprocalOutMax=[]  SumDenOutMin=[]  SumDenOutMax=[]  SumNumOutMin=[]  SumNumOutMax=[]  DivideOutMin=[]  DivideOutMax=[]  UdiffTsProdOutMin=[]  UdiffTsProdOutMax=[]  NTsProdOutMin=[]  NTsProdOutMax=[]  UintegralTsProdOutMin=[]  UintegralTsProdOutMax=[]  UngainTsProdOutMin=[]  UngainTsProdOutMax=[]  ClampingZeroOutDataTypeStr=Inherit: Inherit via back propagation  ClampingZeroOutMin=[]  ClampingZeroOutMax=[]  FilterDenConstantOutDataTypeStr=Inherit: Inherit via back propagation  FilterDenConstantOutMin=[]  FilterDenConstantOutMax=[]  PCopyOutDataTypeStr=Inherit: Inherit via back propagation  PCopyOutMin=[]  PCopyOutMax=[]  NCopyOutDataTypeStr=Inherit: Inherit via back propagation  NCopyOutMin=[]  NCopyOutMax=[]  IntegratorContinuousStateAttributes=''  IntegratorStateMustResolveToSignalObject=off  IntegratorRTWStateStorageClass=Auto  FilterContinuousStateAttributes=''  FilterStateMustResolveToSignalObject=off  FilterRTWStateStorageClass=Auto  ParallelPVariant=InternalParameters  IdealPVariant=Disabled  IVariant=InternalParameters  DVariant=Disabled  IntegratorVariant=Discrete  SatVariant=Enabled  AWVariant=DiscClampingParallel  PCopyVariant=Disabled  TRVariant=Disabled  FdbkBlocksVariant=Forward  IdealPFdbkVariant=Disabled  SatFdbkVariant=Disabled  DerivativeFilterVariant=Disabled  NVariant=Disabled  NCopyVariant=Disabled_SignalSpec  FilterICVariant=Disabled  IntegratorICVariant=InternalICs  ExternalResetVariant=Disabled  TRSumVariant=Passthrough  SumFdbkVariant=Disabled  SumVariant=Sum_PI  TsampFilterVariant=InternalTs  TsampNgainVariant=Passthrough  TsampIntegralVariant=Passthrough  ExternalSaturationOutDataTypeStr=Inherit: Same as second input
  Scope : Scope  NumInputPorts=2
  Scope1 : Scope  NumInputPorts=2
  Sum : Sum  Inputs=|+-
  Sum1 : Sum  Inputs=|+-
  err : Scope  NumInputPorts=2
  ud : Outport
  uq : Outport  Port=2
  wires:
  iq_fdb/1 -> Sum1/2
  Sum1/1 -> PID Controller1/1, err/2  "iq_err"
  id_fdb/1 -> Scope/2, Sum/2
  Sum/1 -> err/1, PID Controller/1  "id_err"
  id_ref/1 -> Scope/1, Sum/1
  iq_ref/1 -> Sum1/1
  PID Controller1/1 -> Scope1/2, uq/1  "uq"
  PID Controller/1 -> Scope1/1, ud/1  "ud"

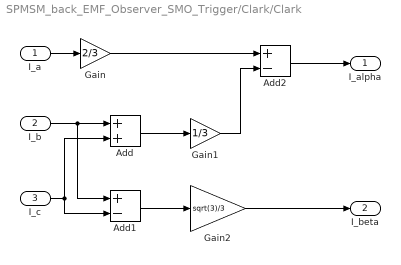
== system SPMSM_back_EMF_Observer_SMO_Trigger/Clark/Clark ==
  I_a : Inport
  I_b : Inport  Port=2
  I_c : Inport  Port=3
  Add : Sum
  Add1 : Sum  Inputs=+-
  Add2 : Sum  Inputs=+-
  Gain : Gain  Gain=2/3
  Gain1 : Gain  Gain=1/3
  Gain2 : Gain  Gain=sqrt(3)/3
  I_alpha : Outport
  I_beta : Outport  Port=2
  wires:
  I_a/1 -> Gain/1
  I_b/1 -> Add1/1, Add/1
  I_c/1 -> Add/2, Add1/2
  Add/1 -> Gain1/1
  Add1/1 -> Gain2/1
  Gain/1 -> Add2/1
  Gain1/1 -> Add2/2
  Add2/1 -> I_alpha/1
  Gain2/1 -> I_beta/1

== matlab function SPMSM_back_EMF_Observer_SMO_Trigger/Theta_scope/MATLAB Function ==
  data: theta input; theta_normalize output
function theta_normalize = fcn(theta)
if (theta > pi)
    theta = theta - 2 * pi;
elseif (theta< -pi)
    theta = theta + 2 * pi;
end
theta_normalize = theta;

== matlab function SPMSM_back_EMF_Observer_SMO_Trigger/Theta_scope/MATLAB Function2 ==
  data: theta input; theta_normalize output
function theta_normalize = fcn(theta)
if (theta > pi)
    theta = theta - 2 * pi;
elseif (theta< -pi)
    theta = theta + 2 * pi;
end
theta_normalize = theta;

== matlab function SPMSM_back_EMF_Observer_SMO_Trigger/Theta_scope/MATLAB Function1 ==
  data: theta input; theta_normalize output
function theta_normalize = fcn(theta)
if (theta > pi)
    theta = theta - 2 * pi;
elseif (theta< -pi)
    theta = theta + 2 * pi;
end
theta_normalize = theta;
